simulink model "DFF1"  (R2014a)
settings: Solver=ode45  StartTime=0.0  StopTime=100  RelTol=1e-3
libraries: commutil2 x2, simulink_extras x1
settings Model: Creator=narayan  LastModifiedBy=narayan
settings OptimizationCC: SimCompilerOptimization=off
settings DebuggingCC: MergeDetectMultiDrivingBlocksExec=error  FrameProcessingCompatibilityMsg=error  AllowSymbolicDim=off
settings RTWCC: RTWCompilerOptimization=off
settings ConfigComp: CovMetricSettings=dw  CovHtmlReporting=on  CovSaveCumulativeToWorkspaceVar=on  CovSaveSingleToWorkspaceVar=on  CovModelRefEnable=Off  CovExternalEMLEnable=off  CovSFcnEnable=off

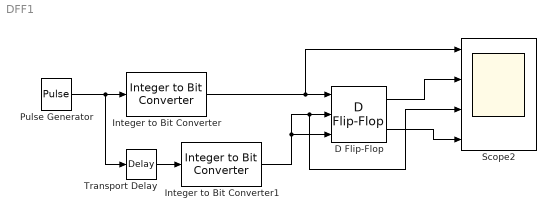
== system DFF1 ==
  D Flip-Flop : simulink_extras/Flip Flops/D Flip-Flop
  Integer to Bit Converter : commutil2/Integer to Bit Converter  nbits=3  signedInputValues=Unsigned  bitOrder=MSB first  outDtype=Inherit via internal rule
  Integer to Bit Converter1 : commutil2/Integer to Bit Converter  nbits=3  signedInputValues=Unsigned  bitOrder=MSB first  outDtype=Inherit via internal rule
  Pulse Generator : DiscretePulseGenerator  Period=7  PulseWidth=5  PhaseDelay=2
  Scope2 : Scope  NumInputPorts=4
      settings: TimeRange=10  YMin=-5~-5~-5~-5  YMax=5~5~5~5
  Transport Delay : TransportDelay  DelayTime=2
  wires:
  Pulse Generator/1 -> Transport Delay/1, Integer to Bit Converter/1
  Integer to Bit Converter/1 -> Scope2/1, D Flip-Flop/1
  Transport Delay/1 -> Integer to Bit Converter1/1
  Integer to Bit Converter1/1 -> D Flip-Flop/3, Scope2/3, D Flip-Flop/2
  D Flip-Flop/1 -> Scope2/2
  D Flip-Flop/2 -> Scope2/4
